simulink model "EarlyReturn10_2018a"  (R2018a)
settings: Solver=VariableStepAuto  StartTime=0.0  StopTime=0.1  RelTol=1e-3
settings Model: Creator=BEAR  LastModifiedBy=bzhan

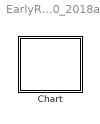
== system EarlyReturn10_2018a ==
  Chart : Stateflow chart  TreatAsAtomicUnit=on

== stateflow chart EarlyReturn10_2018a/Chart ==
  state A
    en: f("en_A")
    ex: f("ex_A")
    state A1
      en: f("en_A1")
      ex: f("ex_A1")
    state A2
      en: f("en_A2")
      ex: f("ex_A2")
    (default) -> A1
    A1 -> (junction 12) : {f("pre");E}
    (junction 12) -> A2 : {f("E")}
  state B
    en: f("en_B")
    ex: f("ex_B")
  (default) -> A
  A -> B : E
  data: s function_input
  events: E local FUNCTION_CALL_EVENT
  function f(s):
    | function f(s)
    |   fprintf(s+"\n");
